simulink model "Heat_pump_model"  (R2020b)
settings: Solver=VariableStepAuto  StartTime=0.0  StopTime=24*60*60  FixedStep=60  RelTol=1e-7
settings Model: Creator=enzlp  LastModifiedBy=enzlp
settings SolverCC: AlgebraicLoopSolver=LineSearch

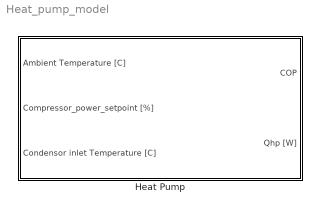
== system Heat_pump_model ==
  Heat Pump : Subsystem

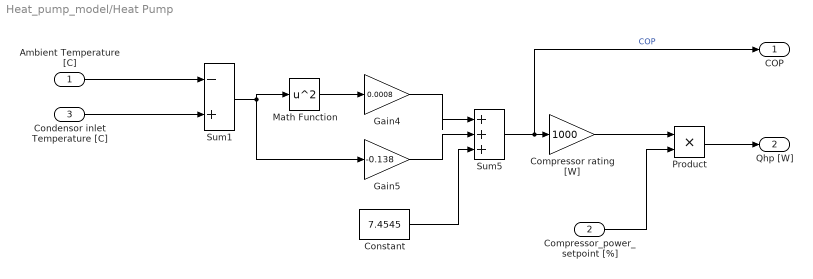
== system Heat_pump_model/Heat Pump ==
  Ambient Temperature [C] : Inport
  Compressor_power_setpoint [%] : Inport  Port=2
  Condensor inlet Temperature [C] : Inport  Port=3
  Compressor rating [W] : Gain  Gain=1000
  Constant : Constant  Value=7.4545
  Gain4 : Gain  Gain=0.0008
  Gain5 : Gain  Gain=-0.138
  Math Function : Math  Operator=square  SignedPower=on  SaturateOnIntegerOverflow=on
  Product : Product
  Sum1 : Sum  Inputs=-+
  Sum5 : Sum  Inputs=|+++
  COP : Outport  VectorParamsAs1DForOutWhenUnconnected=off
  Qhp [W] : Outport  Port=2
  wires:
  Sum1/1 -> Math Function/1, Gain5/1
  Condensor inlet Temperature [C]/1 -> Sum1/2
  Gain4/1 -> Sum5/1
  Constant/1 -> Sum5/3
  Gain5/1 -> Sum5/2
  Sum5/1 -> Compressor rating [W]/1, COP/1  "COP"
  Ambient Temperature [C]/1 -> Sum1/1
  Math Function/1 -> Gain4/1
  Compressor rating [W]/1 -> Product/1
  Product/1 -> Qhp [W]/1
  Compressor_power_setpoint [%]/1 -> Product/2
